simulink model "Driveline_ctrl_sim_con_accion_int"  (R2020a)
settings: Solver=ode45  StartTime=0.0  StopTime=30  MaxStep=0.001  RelTol=1e-3
values from neighbouring files (symbols this model uses):
  A = [[-1/tau 0];[1/m -rho*CD*Af*x2e/m]]    [CruiseCtrl_StateFeedback_Int_design.m]    (also in CruiseCtrl_StateFeedback_Int_design_EJ6.m = Aaug; Driveline_ctrl_design.m = [-ds/(Jf*i^2) ds/(Jf*i) -cs/(Jf*i); Driveline_ctrl_design_accion_int.m = [-ds/(Jf*i^2) ds/(Jf*i) -cs/(Jf*i); active_suspension_ctrl_design.m = [[0 1 0 0 0];[-(cw+cs)/mw -ds/mw cs/mw ds/mw -1/mw];[0 0 0 1)
  B1 = [B H]    [CruiseCtrl_StateFeedback_Int_design.m]    (also in CruiseCtrl_StateFeedback_Int_design_EJ6.m = [Baug Haug]; Driveline_ctrl_design.m; Driveline_ctrl_design_accion_int.m; active_suspension_ctrl_design.m)
  C = [0 1]    [CruiseCtrl_StateFeedback_Int_design.m]    (also in CruiseCtrl_StateFeedback_Int_design_EJ6.m; Driveline_ctrl_design.m = eye(3); Driveline_ctrl_design_accion_int.m = eye(3); active_suspension_ctrl_design.m = [[-1 0 1 0 0];[cs/mc ds/mc -cs/mc -ds/mc 1/mc]])
  D = [0]    [CruiseCtrl_StateFeedback_Int_design.m]    (also in CruiseCtrl_StateFeedback_Int_design_EJ6.m; Driveline_ctrl_design.m = zeros(3,2); Driveline_ctrl_design_accion_int.m = zeros(3,2))
  K = acker(A,B,polos)    [CruiseCtrl_StateFeedback_Int_design.m]    (also in Driveline_ctrl_design.m; Driveline_ctrl_design_accion_int.m = Kaug(1, 1:3); active_suspension_ctrl_design.m = lqr(A,B,Qx,Qu))
  Ki = Kaug(4)    [Driveline_ctrl_design_accion_int.m]
  kr = -1 / X    [CruiseCtrl_StateFeedback_Int_design.m]    (also in Driveline_ctrl_design.m; Driveline_ctrl_design_accion_int.m; active_suspension_ctrl_design.m)
  x0 = [120 2 0]'    [Driveline_ctrl_design.m]    (also in Driveline_ctrl_design_accion_int.m)
settings Model: Creator=jofr  LastModifiedBy=Adriana
settings DataIOCC: LimitDataPoints=on  SaveFormat=Array  SignalLoggingSaveFormat=ModelDataLogs  ReturnWorkspaceOutputs=off
settings OptimizationCC: BlockReduction=off  BooleanDataType=off  LifeSpan=inf
settings DebuggingCC: SaveWithParameterizedLinksMsg=none  UnderspecifiedInitializationDetection=Classic  MergeDetectMultiDrivingBlocksExec=none  SignalResolutionControl=TryResolveAllWithWarning  MultiTaskDSMMsg=warning  MultiTaskCondExecSysMsg=none  SFUnexpectedBacktrackingDiag=warning  SFNoUnconditionalDefaultTransitionDiag=warning  SFExecutionAtInitializationDiag=none  ArithmeticOperatorsInVariantConditions=warning
settings HardwareCC: ProdBitPerPointer=32  ProdBitPerSizeT=32  ProdBitPerPtrDiffT=32  ProdLargestAtomicFloat=None  ProdIntDivRoundTo=Undefined  ProdEndianess=Unspecified  ProdWordSize=32  ProdHWDeviceType=32-bit Generic  TargetUnknown=on
settings ModelReferenceCC: PropagateSignalLabelsOutOfModel=off
settings SFSimCC: SimUseLocalCustomCode=off  CustomCodeUndefinedFunction=UseInterfaceOnly
settings RTWCC: RTWUseLocalCustomCode=off
settings CodeAppCC: StateflowObjectComments=on
settings GRTTargetCC: TargetLangStandard=C89/C90 (ANSI)
settings ConfigComp: CovMetricSettings=dw  CovHtmlReporting=on  CovSaveCumulativeToWorkspaceVar=on  CovSaveSingleToWorkspaceVar=on  CovExternalEMLEnable=off

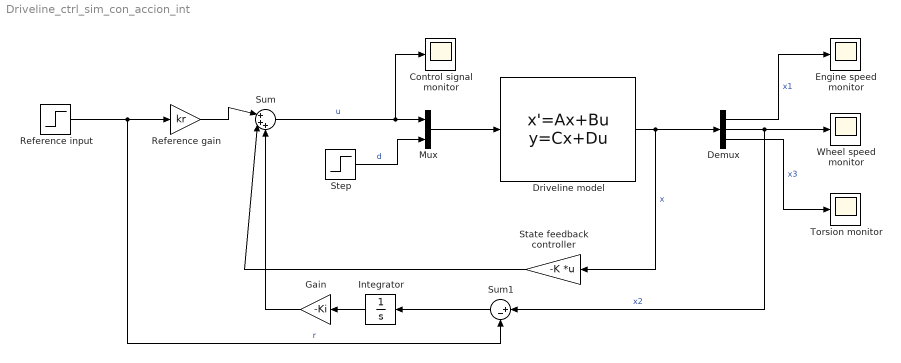
== system Driveline_ctrl_sim_con_accion_int ==
  Control signal monitor : Scope
  Demux : Demux  Outputs=3
  Driveline model : StateSpace  A=A  B=B1  C=C  D=D  InitialCondition=x0
  Engine speed monitor : Scope
  Gain : Gain  Gain=-Ki
  Integrator : Integrator
  Mux : Mux  Inputs=2
  Reference gain : Gain  Gain=kr
  Reference input : Step  Before=2  After=4  SampleTime=0
  State feedback controller : Gain  Gain=-K  Multiplication=Matrix(K*u)
  Step : Step  Time=15  After=10  SampleTime=0
  Sum : Sum  Inputs=|+++
  Sum1 : Sum  Inputs=|+-
  "Torsion monitor " : Scope
  Wheel speed monitor : Scope
  wires:
  Driveline model/1 -> Demux/1, State feedback controller/1  "x"
  Demux/1 -> Engine speed monitor/1  "x1"
  Demux/2 -> Sum1/1, Wheel speed monitor/1  "x2"
  Demux/3 -> "Torsion monitor "/1  "x3"
  Mux/1 -> Driveline model/1
  Step/1 -> Mux/2  "d"
  State feedback controller/1 -> Sum/2
  Reference input/1 -> Sum1/2, Reference gain/1  "r"
  Sum/1 -> Control signal monitor/1, Mux/1  "u"
  Reference gain/1 -> Sum/1
  Sum1/1 -> Integrator/1
  Integrator/1 -> Gain/1
  Gain/1 -> Sum/3
